simulink model "passband_filter"  (R2024b)
settings: Solver=VariableStepAuto  StartTime=0.0  StopTime=11.152  RelTol=1e-3
settings Model: Creator=riccardoorlandi  LastModifiedBy=riccardoorlandi

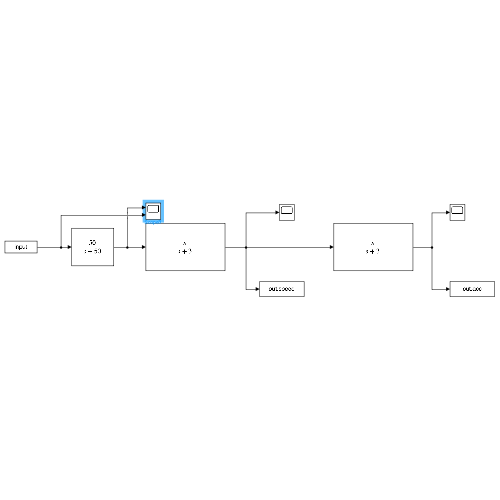
[thumbnail: Simulink's stored preview of the top-level diagram]
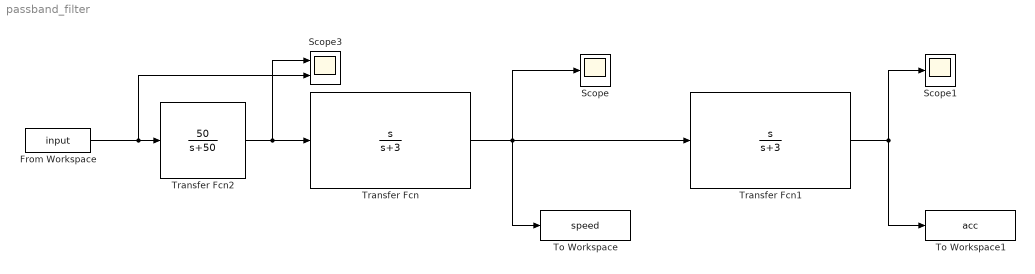
== system passband_filter ==
  From Workspace : FromWorkspace  VariableName=input  SampleTime=0.002
  Scope : Scope
  Scope1 : Scope
  Scope3 : Scope  NumInputPorts=2
  To Workspace : ToWorkspace  VariableName=speed  SampleTime=-1
      settings: Save2DSignal=2-D array (concatenate along first dimension)
  To Workspace1 : ToWorkspace  VariableName=acc  SampleTime=-1
      settings: Save2DSignal=2-D array (concatenate along first dimension)
  Transfer Fcn : TransferFcn  Numerator=[1 0]  Denominator=[1 3]
  Transfer Fcn1 : TransferFcn  Numerator=[1 0]  Denominator=[1 3]
  Transfer Fcn2 : TransferFcn  Numerator=[50]  Denominator=[1 50]
  wires:
  Transfer Fcn/1 -> Transfer Fcn1/1, Scope/1, To Workspace/1
  From Workspace/1 -> Scope3/2, Transfer Fcn2/1
  Transfer Fcn1/1 -> Scope1/1, To Workspace1/1
  Transfer Fcn2/1 -> Scope3/1, Transfer Fcn/1
